simulink model "VCMGCM1962020b_v2"  (R2020b)
settings: Solver=FixedStepDiscrete  StartTime=0.0  StopTime=10.0  FixedStep=0.005  RelTol=1e-3  EnableMultiTasking=on
PreLoadFcn:
  | try, model_open; catch, disp('Error occurred while executing model pre-load callback: model_open.m'); disp('Please assure that the MATLAB working directory is set to the model directory before opening.'); end
InitFcn:
  | try, model_open; catch, end
undefined symbols (not defined in the file): Bridge, GCM, H, raptor_get_param_eval, raptor_get_safe_string, raptor_xcp_function
libraries: Blocks_lib x1165, Raptor_lib x665, simulink x62, VCM_lib x5
(part 13 of 23)

== system VCMGCM1962020b_v2/Fgnd/Sensors/CAN/DC//DC Converter/DCDC_Status_0_16V ==
  DiagEnbl : Inport
  Bus Creator : BusCreator  Inputs=7
  CANRxField1 : Blocks_lib/CANRxField  typ='uint8'  custom=off  custom_nam=[nam '---']  custom_units='---'
  CANRxField2 : Blocks_lib/CANRxField  typ='double'  custom=off  custom_nam=[nam '---']  custom_units='---'
  CANRxField3 : Blocks_lib/CANRxField  typ='double'  custom=off  custom_nam=[nam '---']  custom_units='---'
  CANRxField4 : Blocks_lib/CANRxField  typ='uint16'  custom=off  custom_nam=[nam '---']  custom_units='---'
  CANRxField5 : Blocks_lib/CANRxField  typ='boolean'  custom=off  custom_nam=[nam '---']  custom_units='---'
  CANRxField6 : Blocks_lib/CANRxField  typ='double'  custom=off  custom_nam=[nam '---']  custom_units='---'
  CANRxMsgStatus : Blocks_lib/CANRxMsgStatus  samptime=samptime  custom=off  custom_nam=['---']  msgnam=DCDC_Status_0_16V
  Header : Blocks_lib/Header  width=Landscape  addtext=''
  raptor_can_rxmsg : Raptor_lib/CAN/raptor_can_rxmsg  canDefinition=struct('dbcFile', 'Dilong DCDC Converter_dbc file_v2.dbc','message', 'DCDC_Status_0_16V','comment', '','signals', {{'Fault_alarm2_0_16V','Fault_alarm1_0_16V','DCDC_Output_Current_0_16V','DCDCOutput_Voltage_0_16V','DCDC_Run_status_0_16V','DCDC_Inner_temp_0_16V'}},'enabled', [ 1 1 1 1 1 1;],'scaled', [ 1 1 1 1 1 1;],'canBus', 'bus','messageID', [ 402712053;],'idMask', [ 536870911;],'payloadMask', [],'payloadValue', [],'period', [ 0;],'mailbox', '''''','queueSize', [ 1;],'label', [ 1;],'ver', [ 2;],'showID', [ 0;],'showRaw', [ 0;],'fill', [ 0;],'editID', [ 0;],'signalOrder', [ 3;],'signalAscDes', [ 1;])  canBus=bus  mailbox=''  payloadMask=[]  payloadValue=[]  idMask=hex2dec('1FFFFFFF')  queueSize=1  showID=0  label=1  fill=0  id=402712053  showRaw=0  showAge=1  signalOrder=3  signalInfo={{struct('Name', 'Fault_alarm2_0_16V','Startbit', [ 0;],'SignalSize', [ 8;],'ByteOrder', 'LittleEndian','ValueType', 'UNSIGNED','Class', 'uint8','Signed', [ 0;],'Factor', [ 1;],'Offset', [ 0;],'Min', [ 0;],'Max', [ 128;],'Units', '','Comment', '','StartBit', [ 8;]),struct('Name', 'Fault_alarm1_0_16V','Startbit', [ 0;],'SignalSize', [ 8;],'ByteOrder', 'LittleEndian','ValueType', 'UNSIGNED','Class', 'uint8','Signed', [ 0;],'Factor', [ 1;],'Offset', [ 0;],'Min', [ 0;],'Max', [ 128;],'Units', '','Comment', '','StartBit', [ 16;]),struct('Name', 'DCDC_Output_Current_0_16V','Startbit', [ 0;],'SignalSize', [ 16;],'ByteOrder', 'LittleEndian','ValueType', 'UNSIGNED','Class', 'uint16','Signed', [ 0;],'Factor', [ 0.1;],'Offset', [ 0;],'Min', [ 0;],'Max', [ 1500;],'Units', 'A','Comment', '','StartBit', [ 24;]),struct('Name', 'DCDCOutput_Voltage_0_16V','Startbit', [ 0;],'SignalSize', [ 8;],'ByteOrder', 'LittleEndian','ValueType', 'UNSIGNED','Class', 'uint8','Signed', [ 0;],'Factor', [ 0.2;],'Offset', [ 0;],'Min', [ 0;],'Max', [ 150;],'Units', 'V','Comment', '','StartBit', [ 40;]),struct('Name', 'DCDC_Run_status_0_16V','Startbit', [ 0;],'SignalSize', [ 1;],'ByteOrder', 'LittleEndian','ValueType', 'UNSIGNED','Class', 'uint8','Signed', [ 0;],'Factor', [ 1;],'Offset', [ 0;],'Min', [ 0;],'Max', [ 1;],'Units', '','Comment', '','StartBit', [ 48;]),struct('Name', 'DCDC_Inner_temp_0_16V','Startbit', [ 0;],'SignalSize', [ 8;],'ByteOrder', 'LittleEndian','ValueType', 'UNSIGNED','Class', 'uint8','Signed', [ 0;],'Factor', [ 1;],'Offset', [ -40;],'Min', [ 0;],'Max', [ 128;],'Units', 'C','Comment', '','StartBit', [ 56;])}}
      settings: SourceProductName=Raptor
  Data : Outport  VectorParamsAs1DForOutWhenUnconnected=off
  wires:
  Bus Creator/1 -> Data/1  "DCDC_Status_0_16V"
  raptor_can_rxmsg/2 -> CANRxField4/1  "Fault_alarm2_0_16V"
  raptor_can_rxmsg/3 -> CANRxField1/1  "Fault_alarm1_0_16V"
  raptor_can_rxmsg/4 -> CANRxField3/1  "DCDC_Output_Current_0_16V"
  DiagEnbl/1 -> CANRxMsgStatus/1
  raptor_can_rxmsg/1 -> CANRxMsgStatus/2  "Age"
  CANRxMsgStatus/1 -> Bus Creator/1
  CANRxField4/1 -> Bus Creator/2
  CANRxField1/1 -> Bus Creator/3
  CANRxField3/1 -> Bus Creator/4
  CANRxField2/1 -> Bus Creator/7
  raptor_can_rxmsg/7 -> CANRxField2/1  "DCDC_Inner_temp_0_16V"
  raptor_can_rxmsg/6 -> CANRxField5/1  "DCDC_Run_status_0_16V"
  raptor_can_rxmsg/5 -> CANRxField6/1  "DCDCOutput_Voltage_0_16V"
  CANRxField5/1 -> Bus Creator/6
  CANRxField6/1 -> Bus Creator/5

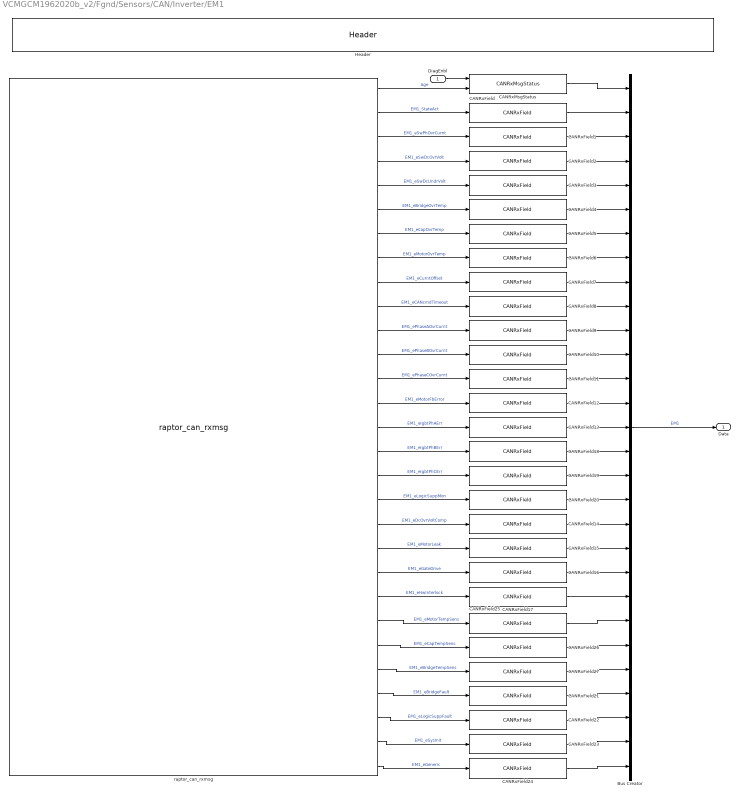
== system VCMGCM1962020b_v2/Fgnd/Sensors/CAN/Inverter/EM1 ==
  DiagEnbl : Inport
  Bus Creator : BusCreator  Inputs=29
  CANRxField : Blocks_lib/CANRxField  typ='uint8'  custom=off  custom_nam='---'  custom_units='---'
  CANRxField{1..24,26..27} (26 alike) : Blocks_lib/CANRxField  typ='boolean'  custom=off  custom_nam='---'  custom_units='---'
  CANRxField25 : Blocks_lib/CANRxField  typ='uint8'  custom=off  custom_nam='---'  custom_units='---'
  CANRxMsgStatus : Blocks_lib/CANRxMsgStatus  samptime=samptime  custom=off  custom_nam='Name'  msgnam=EM1
  Header : Blocks_lib/Header  width=Landscape  addtext=''
  raptor_can_rxmsg : Raptor_lib/CAN/raptor_can_rxmsg  canDefinition=struct('dbcFile', '20220526e_emDrive_NodeID_0x01.dbc','message', 'EM1','comment', '100ms','signals', {{'EM1_StateAct','EM1_eSwPhOvrCurnt','EM1_eSwDcOvrVolt','EM1_eSwDcUndrVolt','EM1_eBridgeOvrTemp','EM1_eCapOvrTemp','EM1_eMotorOvrTemp','EM1_eCurntOffset','EM1_eCANcmdTimeout','EM1_ePhaseAOvrCurnt','EM1_ePhaseBOvrCurnt','EM1_ePhaseCOvrCurnt','EM1_eMotorFbError','EM1_eIgbtPhAErr','EM1_eIgbtPhBErr','EM1_eIgbtPhCErr','EM1_eLogicSuppMon','EM1_eDcOvrVoltComp','EM1_eMotorLeak','EM1_eGateDrive','EM1_eHwInterlock','EM1_eMotorTempSens','EM1_eCapTempSens','EM1_eBridgeTempSens','EM1_eBridgeFault','EM1_eLogicSuppFault','EM1_eSysInit','EM1_eGeneric'}},'enabled', [ 1 1 1 1 1 1 1 1 1 1 1 1 1 1 1 1 1 1 1 1 1 1 1 1 1 1 1 1;],'scaled', [ 1 1 1 1 1 1 1 1 1 1 1 1 1 1 1 1 1 1 1 1 1 1 1 1 1 1 1 1;],'canBus', 'bus','messageID', [ 385;],'idMask', [ 536870911;],'payloadMask', [],'payloadValue', [],'period', [ 0;],'mailbox', '''''','queueSize', [ 1;],'label', [ 1;],'ver', [ 2;],'showID', [ 0;],'showRaw', [ 0;],'showRawMsg', [ 0;],'showAge', [ 1;],'fill', [ 0;],'editID', [ 0;],'signalOrder', [ 3;],'signalAscDes', [ 1;])  canBus=bus  mailbox=''  payloadMask=[]  payloadValue=[]  idMask=hex2dec('1FFFFFFF')  queueSize=1  showID=0  label=1  fill=0  id=385  showRaw=0  showAge=1  signalOrder=3  signalInfo={{struct('Name', 'EM1_StateAct','Startbit', [ 0;],'SignalSize', [ 8;],'ByteOrder', 'LittleEndian','ValueType', 'UNSIGNED','Class', 'uint8','Signed', [ 0;],'Factor', [ 1;],'Offset', [ 0;],'Min', [ -2;],'Max', [ 2;],'Units', '','Comment', 'Application_Control__State','StartBit', [ 0;]),struct('Name', 'EM1_eSwPhOvrCurnt','Startbit', [ 0;],'SignalSize', [ 1;],'ByteOrder', 'LittleEndian','ValueType', 'UNSIGNED','Class', 'uint8','Signed', [ 0;],'Factor', [ 1;],'Offset', [ 0;],'Min', [ 0;],'Max', [ 1;],'Units', '','Comment', 'Software phase overcurrent','StartBit', [ 8;]),struct('Name', 'EM1_eSwDcOvrVolt','Startbit', [ 0;],'SignalSize', [ 1;],'ByteOrder', 'LittleEndian','ValueType', 'UNSIGNED','Class', 'uint8','Signed', [ 0;],'Factor', [ 1;],'Offset', [ 0;],'Min', [ 0;],'Max', [ 1;],'Units', '','Comment', 'Software DC link overvoltage','StartBit', [ 9;]),struct('Name', 'EM1_eSwDcUndrVolt','Startbit', [ 0;],'SignalSize', [ 1;],'ByteOrder', 'LittleEndian','ValueType', 'UNSIGNED','Class', 'uint8','Signed', [ 0;],'Factor', [ 1;],'Offset', [ 0;],'Min', [ 0;],'Max', [ 1;],'Units', '','Comment', 'Software DC link undervoltage','StartBit', [ 10;]),struct('Name', 'EM1_eBridgeOvrTemp','Startbit', [ 0;],'SignalSize', [ 1;],'ByteOrder', 'LittleEndian','ValueType', 'UNSIGNED','Class', 'uint8','Signed', [ 0;],'Factor', [ 1;],'Offset', [ 0;],'Min', [ 0;],'Max', [ 1;],'Units', '','Comment', 'Bridge overtemperature','StartBit', [ 11;]),struct('Name', 'EM1_eCapOvrTemp','Startbit', [ 0;],'SignalSize', [ 1;],'ByteOrder', 'LittleEndian','ValueType', 'UNSIGNED','Class', 'uint8','Signed', [ 0;],'Factor', [ 1;],'Offset', [ 0;],'Min', [ 0;],'Max', [ 1;],'Units', '','Comment', 'Capacitor overtemperature','StartBit', [ 12;]),struct('Name', 'EM1_eMotorOvrTemp','Startbit', [ 0;],'SignalSize', [ 1;],'ByteOrder', 'LittleEndian','ValueType', 'UNSIGNED','Class', 'uint8','Signed', [ 0;],'Factor', [ 1;],'Offset', [ 0;],'Min', [ 0;],'Max', [ 1;],'Units', '','Comment', 'Motor overtemperature','StartBit', [ 13;]),struct('Name', 'EM1_eCurntOffset','Startbit', [ 0;],'SignalSize', [ 1;],'ByteOrder', 'LittleEndian','ValueType', 'UNSIGNED','Class', 'uint8','Signed', [ 0;],'Factor', [ 1;],'Offset', [ 0;],'Min', [ 0;],'Max', [ 1;],'Units', '','Comment', 'Current offset','StartBit', [ 14;]),struct('Name', 'EM1_eCANcmdTimeout','Startbit', [ 0;],'SignalSize', [ 1;],'ByteOrder', 'LittleEndian','ValueType', 'UNSIGNED','Class', 'uint8','Signed', [ 0;],'Factor', [ 1;],'Offset', [ 0;],'Min', [ 0;],'Max', [ 1;],'Units', '','Comment', 'CAN Command timeout','StartBit', [ 15;]),struct('Name', 'EM1_ePhaseAOvrCurnt','Startbit', [ 0;],'SignalSize', [ 1;],'ByteOrder', 'LittleEndian','ValueType', 'UNSIGNED','Class', 'uint8','Signed', [ 0;],'Factor', [ 1;],'Offset', [ 0;],'Min', [ 0;],'Max', [ 1;],'Units', '','Comment', 'Phase A overcurrent','StartBit', [ 16;]),struct('Name', 'EM1_ePhaseBOvrCurnt','Startbit', [ 0;],'SignalSize', [ 1;],'ByteOrder', 'LittleEndian','ValueType', 'UNSIGNED','Class', 'uint8','Signed', [ 0;],'Factor', [ 1;],'Offset', [ 0;],'Min', [ 0;],'Max', [ 1;],'Units', '','Comment', 'Phase B overcurrent','StartBit', [ 17;]),struct('Name', 'EM1_ePhaseCOvrCurnt','Startbit', [ 0;],'SignalSize', [ 1;],'ByteOrder', 'LittleEndian','ValueType', 'UNSIGNED','Class', 'uint8','Signed', [ 0;],'Factor', [ 1;],'Offset', [ 0;],'Min', [ 0;],'Max', [ 1;],'Units', '','Comment', 'Phase C overcurrent','StartBit', [ 18;]),struct('Name', 'EM1_eMotorFbError','Startbit', [ 0;],'SignalSize', [ 1;],'ByteOrder', 'LittleEndian','ValueType', 'UNSIGNED','Class', 'uint8','Signed', [ 0;],'Factor', [ 1;],'Offset', [ 0;],'Min', [ 0;],'Max', [ 1;],'Units', '','Comment', 'Motor feedback error','StartBit', [ 19;]),struct('Name', 'EM1_eIgbtPhAErr','Startbit', [ 0;],'SignalSize', [ 1;],'ByteOrder', 'LittleEndian','ValueType', 'UNSIGNED','Class', 'uint8','Signed', [ 0;],'Factor', [ 1;],'Offset', [ 0;],'Min', [ 0;],'Max', [ 1;],'Units', '','Comment', 'IGBT Phase A error','StartBit', [ 20;]),struct('Name', 'EM1_eIgbtPhBErr','Startbit', [ 0;],'SignalSize', [ 1;],'ByteOrder', 'LittleEndian','ValueType', 'UNSIGNED','Class', 'uint8','Signed', [ 0;],'Factor', [ 1;],'Offset', [ 0;],'Min', [ 0;],'Max', [ 1;],'Units', '','Comment', 'IGBT Phase B error','StartBit', [ 21;]),struct('Name', 'EM1_eIgbtPhCErr','Startbit', [ 0;],'SignalSize', [ 1;],'ByteOrder', 'LittleEndian','ValueType', 'UNSIGNED','Class', 'uint8','Signed', [ 0;],'Factor', [ 1;],'Offset', [ 0;],'Min', [ 0;],'Max', [ 1;],'Units', '','Comment', 'IGBT Phase C error','StartBit', [ 22;]),struct('Name', 'EM1_eLogicSuppMon','Startbit', [ 0;],'SignalSize', [ 1;],'ByteOrder', 'LittleEndian','ValueType', 'UNSIGNED','Class', 'uint8','Signed', [ 0;],'Factor', [ 1;],'Offset', [ 0;],'Min', [ 0;],'Max', [ 1;],'Units', '','Comment', 'Logic Supply monitor error','StartBit', [ 24;]),struct('Name', 'EM1_eDcOvrVoltComp','Startbit', [ 0;],'SignalSize', [ 1;],'ByteOrder', 'LittleEndian','ValueType', 'UNSIGNED','Class', 'uint8','Signed', [ 0;],'Factor', [ 1;],'Offset', [ 0;],'Min', [ 0;],'Max', [ 1;],'Units', '','Comment', 'DC link overvoltage comparator','StartBit', [ 25;]),struct('Name', 'EM1_eMotorLeak','Startbit', [ 0;],'SignalSize', [ 1;],'ByteOrder', 'LittleEndian','ValueType', 'UNSIGNED','Class', 'uint8','Signed', [ 0;],'Factor', [ 1;],'Offset', [ 0;],'Min', [ 0;],'Max', [ 1;],'Units', '','Comment', 'Motor leakage','StartBit', [ 26;]),struct('Name', 'EM1_eGateDrive','Startbit', [ 0;],'SignalSize', [ 1;],'ByteOrder', 'LittleEndian','ValueType', 'UNSIGNED','Class', 'uint8','Signed', [ 0;],'Factor', [ 1;],'Offset', [ 0;],'Min', [ 0;],'Max', [ 1;],'Units', '','Comment', 'Gatedriver error','StartBit', [ 27;]),struct('Name', 'EM1_eHwInterlock','Startbit', [ 0;],'SignalSize', [ 1;],'ByteOrder', 'LittleEndian','ValueType', 'UNSIGNED','Class', 'uint8','Signed', [ 0;],'Factor', [ 1;],'Offset', [ 0;],'Min', [ 0;],'Max', [ 1;],'Units', '','Comment', 'HW interlock','StartBit', [ 28;]),struct('Name', 'EM1_eMotorTempSens','Startbit', [ 0;],'SignalSize', [ 1;],'ByteOrder', 'LittleEndian','ValueType', 'UNSIGNED','Class', 'uint8','Signed', [ 0;],'Factor', [ 1;],'Offset', [ 0;],'Min', [ 0;],'Max', [ 1;],'Units', '','Comment', 'Motor temperature sensor fail','StartBit', [ 29;]),struct('Name', 'EM1_eCapTempSens','Startbit', [ 0;],'SignalSize', [ 1;],'ByteOrder', 'LittleEndian','ValueType', 'UNSIGNED','Class', 'uint8','Signed', [ 0;],'Factor', [ 1;],'Offset', [ 0;],'Min', [ 0;],'Max', [ 1;],'Units', '','Comment', 'Capacitor temperature sensor fail','StartBit', [ 30;]),struct('Name', 'EM1_eBridgeTempSens','Startbit', [ 0;],'SignalSize', [ 1;],'ByteOrder', 'LittleEndian','ValueType', 'UNSIGNED','Class', 'uint8','Signed', [ 0;],'Factor', [ 1;],'Offset', [ 0;],'Min', [ 0;],'Max', [ 1;],'Units', '','Comment', 'Bridge temperature sensor fail','StartBit', [ 31;]),struct('Name', 'EM1_eBridgeFault','Startbit', [ 0;],'SignalSize', [ 1;],'ByteOrder', 'LittleEndian','ValueType', 'UNSIGNED','Class', 'uint8','Signed', [ 0;],'Factor', [ 1;],'Offset', [ 0;],'Min', [ 0;],'Max', [ 1;],'Units', '','Comment', 'Bridge fault (check BridgeFault object for details)','StartBit', [ 32;]),struct('Name', 'EM1_eLogicSuppFault','Startbit', [ 0;],'SignalSize', [ 1;],'ByteOrder', 'LittleEndian','ValueType', 'UNSIGNED','Class', 'uint8','Signed', [ 0;],'Factor', [ 1;],'Offset', [ 0;],'Min', [ 0;],'Max', [ 1;],'Units', '','Comment', 'Logic supply fault','StartBit', [ 33;]),struct('Name', 'EM1_eSysInit','Startbit', [ 0;],'SignalSize', [ 1;],'ByteOrder', 'LittleEndian','ValueType', 'UNSIGNED','Class', 'uint8','Signed', [ 0;],'Factor', [ 1;],'Offset', [ 0;],'Min', [ 0;],'Max', [ 1;],'Units', '','Comment', 'System initialization error','StartBit', [ 38;]),struct('Name', 'EM1_eGeneric','Startbit', [ 0;],'SignalSize', [ 1;],'ByteOrder', 'LittleEndian','ValueType', 'UNSIGNED','Class', 'uint8','Signed', [ 0;],'Factor', [ 1;],'Offset', [ 0;],'Min', [ 0;],'Max', [ 1;],'Units', '','Comment', 'Generic error','StartBit', [ 39;])}}
      settings: SourceProductName=Raptor
  Data : Outport  VectorParamsAs1DForOutWhenUnconnected=off
  wires:
  Bus Creator/1 -> Data/1  "EM1"
  raptor_can_rxmsg/2 -> CANRxField/1  "EM1_StateAct"
  CANRxMsgStatus/1 -> Bus Creator/1
  DiagEnbl/1 -> CANRxMsgStatus/1
  raptor_can_rxmsg/1 -> CANRxMsgStatus/2  "Age"
  raptor_can_rxmsg/3 -> CANRxField1/1  "EM1_eSwPhOvrCurnt"
  raptor_can_rxmsg/4 -> CANRxField2/1  "EM1_eSwDcOvrVolt"
  raptor_can_rxmsg/5 -> CANRxField3/1  "EM1_eSwDcUndrVolt"
  raptor_can_rxmsg/6 -> CANRxField4/1  "EM1_eBridgeOvrTemp"
  raptor_can_rxmsg/7 -> CANRxField5/1  "EM1_eCapOvrTemp"
  raptor_can_rxmsg/8 -> CANRxField6/1  "EM1_eMotorOvrTemp"
  raptor_can_rxmsg/9 -> CANRxField7/1  "EM1_eCurntOffset"
  raptor_can_rxmsg/10 -> CANRxField8/1  "EM1_eCANcmdTimeout"
  raptor_can_rxmsg/11 -> CANRxField9/1  "EM1_ePhaseAOvrCurnt"
  raptor_can_rxmsg/12 -> CANRxField10/1  "EM1_ePhaseBOvrCurnt"
  raptor_can_rxmsg/13 -> CANRxField11/1  "EM1_ePhaseCOvrCurnt"
  raptor_can_rxmsg/14 -> CANRxField12/1  "EM1_eMotorFbError"
  raptor_can_rxmsg/15 -> CANRxField13/1  "EM1_eIgbtPhAErr"
  raptor_can_rxmsg/16 -> CANRxField18/1  "EM1_eIgbtPhBErr"
  raptor_can_rxmsg/17 -> CANRxField19/1  "EM1_eIgbtPhCErr"
  raptor_can_rxmsg/18 -> CANRxField20/1  "EM1_eLogicSuppMon"
  raptor_can_rxmsg/19 -> CANRxField14/1  "EM1_eDcOvrVoltComp"
  raptor_can_rxmsg/20 -> CANRxField15/1  "EM1_eMotorLeak"
  raptor_can_rxmsg/21 -> CANRxField16/1  "EM1_eGateDrive"
  raptor_can_rxmsg/22 -> CANRxField17/1  "EM1_eHwInterlock"
  raptor_can_rxmsg/23 -> CANRxField25/1  "EM1_eMotorTempSens"
  raptor_can_rxmsg/24 -> CANRxField26/1  "EM1_eCapTempSens"
  raptor_can_rxmsg/25 -> CANRxField27/1  "EM1_eBridgeTempSens"
  raptor_can_rxmsg/26 -> CANRxField21/1  "EM1_eBridgeFault"
  raptor_can_rxmsg/27 -> CANRxField22/1  "EM1_eLogicSuppFault"
  raptor_can_rxmsg/28 -> CANRxField23/1  "EM1_eSysInit"
  raptor_can_rxmsg/29 -> CANRxField24/1  "EM1_eGeneric"
  CANRxField/1 -> Bus Creator/2
  CANRxField1/1 -> Bus Creator/3
  CANRxField2/1 -> Bus Creator/4
  CANRxField3/1 -> Bus Creator/5
  CANRxField4/1 -> Bus Creator/6
  CANRxField5/1 -> Bus Creator/7
  CANRxField6/1 -> Bus Creator/8
  CANRxField7/1 -> Bus Creator/9
  CANRxField8/1 -> Bus Creator/10
  CANRxField9/1 -> Bus Creator/11
  CANRxField10/1 -> Bus Creator/12
  CANRxField11/1 -> Bus Creator/13
  CANRxField12/1 -> Bus Creator/14
  CANRxField13/1 -> Bus Creator/15
  CANRxField18/1 -> Bus Creator/16
  CANRxField19/1 -> Bus Creator/17
  CANRxField20/1 -> Bus Creator/18
  CANRxField14/1 -> Bus Creator/19
  CANRxField15/1 -> Bus Creator/20
  CANRxField16/1 -> Bus Creator/21
  CANRxField17/1 -> Bus Creator/22
  CANRxField25/1 -> Bus Creator/23
  CANRxField26/1 -> Bus Creator/24
  CANRxField27/1 -> Bus Creator/25
  CANRxField21/1 -> Bus Creator/26
  CANRxField22/1 -> Bus Creator/27
  CANRxField23/1 -> Bus Creator/28
  CANRxField24/1 -> Bus Creator/29

== system VCMGCM1962020b_v2/Fgnd/Sensors/CAN/Inverter/EM2_InvTemp ==
  note: This is a CANR Rx structure that was implemented to overcome a error in the way the floating point data was handled. It is not Ideal but does work.
  DiagEnbl : Inport
  Bus Creator1 : BusCreator  Inputs=2
  Bus Creator2 : BusCreator  Inputs=2
  Bus Creator3 : BusCreator  Inputs=2
  Delay : Delay  DelayLength=5
  EM2InvTemp : Subsystem
  EM2MtrTemp : Subsystem
  Header : Blocks_lib/Header  width=Landscape  addtext=''
  NOT : Logic  Operator=NOT  AllPortsSameDT=off  OutDataTypeStr=boolean
  Output : Outport
  wires:
  EM2MtrTemp/1(MsgVld) -> Bus Creator2/1
  EM2MtrTemp/2(Out2) -> Bus Creator2/2
  DiagEnbl/1 -> EM2MtrTemp/1(DiagEnbl), EM2InvTemp/1(DiagEnbl)
  Bus Creator2/1 -> Bus Creator1/2  "EM2MtrTemp"
  Delay/1 -> NOT/1, EM2InvTemp/Enable
  NOT/1 -> Delay/1, EM2MtrTemp/Enable
  Bus Creator1/1 -> Output/1  "EM2"
  EM2InvTemp/1(MsgVld) -> Bus Creator3/1
  EM2InvTemp/2(Out2) -> Bus Creator3/2
  Bus Creator3/1 -> Bus Creator1/1  "EM2Invemp"

== system VCMGCM1962020b_v2/Fgnd/Sensors/CAN/Inverter/EM3 ==
  DiagEnbl : Inport
  Bus Creator : BusCreator  Inputs=3
  CANRxField : Blocks_lib/CANRxField  typ='double'  custom=off  custom_nam='---'  custom_units='---'
  CANRxField1 : Blocks_lib/CANRxField  typ='double'  custom=off  custom_nam='---'  custom_units='---'
  CANRxMsgStatus : Blocks_lib/CANRxMsgStatus  samptime=samptime  custom=off  custom_nam='Name'  msgnam=EM3
  Header : Blocks_lib/Header  width=Landscape  addtext=''
  raptor_can_rxmsg : Raptor_lib/CAN/raptor_can_rxmsg  canDefinition=struct('dbcFile', '20220526e_emDrive_NodeID_0x01.dbc','message', 'EM3','comment', '40ms','signals', {{'EM3_InverterDcV','EM3_PhaseAmpsRms'}},'enabled', [ 1 1;],'scaled', [ 1 1;],'canBus', 'bus','messageID', [ 897;],'idMask', [ 536870911;],'payloadMask', [],'payloadValue', [],'period', [ 0;],'mailbox', '''''','queueSize', [ 1;],'label', [ 1;],'ver', [ 2;],'showID', [ 0;],'showRaw', [ 0;],'fill', [ 0;],'editID', [ 0;],'signalOrder', [ 3;],'signalAscDes', [ 1;])  canBus=bus  mailbox=''  payloadMask=[]  payloadValue=[]  idMask=hex2dec('1FFFFFFF')  queueSize=1  showID=0  label=1  fill=0  id=897  showRaw=0  showAge=1  signalOrder=3  signalInfo={{struct('Name', 'EM3_InverterDcV','Startbit', [ 0;],'SignalSize', [ 32;],'ByteOrder', 'LittleEndian','ValueType', 'FLOAT32','Class', 'single','Signed', [ 1;],'Factor', [ 1;],'Offset', [ 0;],'Min', [ 0;],'Max', [ 0;],'Units', 'V','Comment', 'HW_Monitor__UDC','StartBit', [ 0;]),struct('Name', 'EM3_PhaseAmpsRms','Startbit', [ 0;],'SignalSize', [ 32;],'ByteOrder', 'LittleEndian','ValueType', 'FLOAT32','Class', 'single','Signed', [ 1;],'Factor', [ 1;],'Offset', [ 0;],'Min', [ 0;],'Max', [ 0;],'Units', 'A','Comment', 'HW_Monitor__Phase_Current','StartBit', [ 32;])}}
      settings: SourceProductName=Raptor
  Data : Outport  VectorParamsAs1DForOutWhenUnconnected=off
  wires:
  Bus Creator/1 -> Data/1  "MsgName"
  raptor_can_rxmsg/2 -> CANRxField/1  "EM3_InverterDcV"
  CANRxMsgStatus/1 -> Bus Creator/1
  DiagEnbl/1 -> CANRxMsgStatus/1
  raptor_can_rxmsg/1 -> CANRxMsgStatus/2  "Age"
  CANRxField/1 -> Bus Creator/2
  raptor_can_rxmsg/3 -> CANRxField1/1  "EM3_PhaseAmpsRms"
  CANRxField1/1 -> Bus Creator/3

== system VCMGCM1962020b_v2/Fgnd/Sensors/CAN/Inverter/EM3_DCV ==
  note: This is a CANR Rx structure that was implemented to overcome a error in the way the floating point data was handled. It is not Ideal but does work.
  DiagEnbl : Inport
  Bus Creator1 : BusCreator  Inputs=2
  Bus Creator2 : BusCreator  Inputs=2
  Bus Creator3 : BusCreator  Inputs=2
  Delay : Delay  DelayLength=5
  EM3DCv : Subsystem
  EM3PhCur : Subsystem
  Header : Blocks_lib/Header  width=Landscape  addtext=''
  NOT : Logic  Operator=NOT  AllPortsSameDT=off  OutDataTypeStr=boolean
  Output : Outport
  wires:
  EM3PhCur/1(MsgVld) -> Bus Creator2/1
  EM3PhCur/2(Out2) -> Bus Creator2/2
  DiagEnbl/1 -> EM3PhCur/1(DiagEnbl), EM3DCv/1(DiagEnbl)
  Bus Creator2/1 -> Bus Creator1/2  "EM3PhCur"
  Delay/1 -> NOT/1, EM3DCv/Enable
  NOT/1 -> Delay/1, EM3PhCur/Enable
  Bus Creator1/1 -> Output/1  "EM3"
  EM3DCv/1(MsgVld) -> Bus Creator3/1
  EM3DCv/2(Out2) -> Bus Creator3/2
  Bus Creator3/1 -> Bus Creator1/1  "EM3DCv"

== system VCMGCM1962020b_v2/Fgnd/Sensors/CAN/Inverter/EM4 ==
  DiagEnbl : Inport
  Bus Creator : BusCreator  Inputs=3
  CANRxField : Blocks_lib/CANRxField  typ='double'  custom=off  custom_nam='---'  custom_units='---'
  CANRxField1 : Blocks_lib/CANRxField  typ='double'  custom=off  custom_nam='---'  custom_units='---'
  CANRxMsgStatus : Blocks_lib/CANRxMsgStatus  samptime=samptime  custom=off  custom_nam='Name'  msgnam=EM4
  Header : Blocks_lib/Header  width=Landscape  addtext=''
  raptor_can_rxmsg : Raptor_lib/CAN/raptor_can_rxmsg  canDefinition=struct('dbcFile', '20220526e_emDrive_NodeID_0x01.dbc','message', 'EM4','comment', '20ms','signals', {{'EM4_TorqAct','EM4_SpdAct'}},'enabled', [ 1 1;],'scaled', [ 1 1;],'canBus', 'bus','messageID', [ 641;],'idMask', [ 536870911;],'payloadMask', [],'payloadValue', [],'period', [ 0;],'mailbox', '''''','queueSize', [ 1;],'label', [ 1;],'ver', [ 2;],'showID', [ 0;],'showRaw', [ 0;],'fill', [ 0;],'editID', [ 0;],'signalOrder', [ 3;],'signalAscDes', [ 1;])  canBus=bus  mailbox=''  payloadMask=[]  payloadValue=[]  idMask=hex2dec('1FFFFFFF')  queueSize=1  showID=0  label=1  fill=0  id=641  showRaw=0  showAge=1  signalOrder=3  signalInfo={{struct('Name', 'EM4_TorqAct','Startbit', [ 0;],'SignalSize', [ 32;],'ByteOrder', 'LittleEndian','ValueType', 'FLOAT32','Class', 'single','Signed', [ 1;],'Factor', [ 1;],'Offset', [ 0;],'Min', [ 0;],'Max', [ 0;],'Units', 'Nm','Comment', 'Ctrl_Gen_Stat__Tact','StartBit', [ 0;]),struct('Name', 'EM4_SpdAct','Startbit', [ 0;],'SignalSize', [ 32;],'ByteOrder', 'LittleEndian','ValueType', 'FLOAT32','Class', 'single','Signed', [ 1;],'Factor', [ 1;],'Offset', [ 0;],'Min', [ 0;],'Max', [ 0;],'Units', 'rpm','Comment', 'Ctrl_Gen_Stat__RPMact','StartBit', [ 32;])}}
      settings: SourceProductName=Raptor
  Data : Outport  VectorParamsAs1DForOutWhenUnconnected=off
  wires:
  CANRxField/1 -> Bus Creator/2
  raptor_can_rxmsg/1 -> CANRxMsgStatus/2  "Age"
  DiagEnbl/1 -> CANRxMsgStatus/1
  CANRxMsgStatus/1 -> Bus Creator/1
  raptor_can_rxmsg/2 -> CANRxField/1  "EM4_TorqAct"
  Bus Creator/1 -> Data/1  "MsgName"
  raptor_can_rxmsg/3 -> CANRxField1/1  "EM4_SpdAct"
  CANRxField1/1 -> Bus Creator/3

== system VCMGCM1962020b_v2/Fgnd/Sensors/CAN/Inverter/EM4_Spd ==
  note: This is a CANR Rx structure that was implemented to overcome a error in the way the floating point data was handled. It is not Ideal but does work.
  DiagEnbl : Inport
  Bus Creator1 : BusCreator  Inputs=2
  Bus Creator2 : BusCreator  Inputs=2
  Bus Creator3 : BusCreator  Inputs=2
  Delay : Delay
  EM4Spd : Subsystem
  EM4Torq : Subsystem
  Header : Blocks_lib/Header  width=Landscape  addtext=''
  NOT : Logic  Operator=NOT  AllPortsSameDT=off  OutDataTypeStr=boolean
  Output : Outport
  wires:
  EM4Torq/1(MsgVld) -> Bus Creator2/1
  EM4Torq/2(Out2) -> Bus Creator2/2
  DiagEnbl/1 -> EM4Torq/1(DiagEnbl), EM4Spd/1(DiagEnbl)
  Bus Creator2/1 -> Bus Creator1/2  "EM4Trq"
  Delay/1 -> NOT/1, EM4Spd/Enable
  NOT/1 -> Delay/1, EM4Torq/Enable
  Bus Creator1/1 -> Output/1  "EM4"
  EM4Spd/1(MsgVld) -> Bus Creator3/1
  EM4Spd/2(Out2) -> Bus Creator3/2
  Bus Creator3/1 -> Bus Creator1/1  "EM4Spd"

== system VCMGCM1962020b_v2/Fgnd/Sensors/CAN/Inverter/EM_BOOT ==
  DiagEnbl : Inport
  Bus Creator : BusCreator  Inputs=2
  CANRxField : Blocks_lib/CANRxField  typ='double'  custom=off  custom_nam='---'  custom_units='---'
  CANRxMsgStatus : Blocks_lib/CANRxMsgStatus  samptime=samptime  custom=off  custom_nam='Name'  msgnam=EM_BOOT
  Header : Blocks_lib/Header  width=Landscape  addtext=''
  raptor_can_rxmsg : Raptor_lib/CAN/raptor_can_rxmsg  canDefinition=struct('dbcFile', '20220526e_emDrive_NodeID_0x01.dbc','message', 'EM_BOOT','comment', 'Sent after boot has completed and comms are available','signals', {{'EM_BOOT_EmBoot'}},'enabled', [ 1;],'scaled', [ 1;],'canBus', 'bus','messageID', [ 1793;],'idMask', [ 536870911;],'payloadMask', [],'payloadValue', [],'period', [ 0;],'mailbox', '''''','queueSize', [ 1;],'label', [ 1;],'ver', [ 2;],'showID', [ 0;],'showRaw', [ 0;],'showRawMsg', [ 0;],'showAge', [ 1;],'fill', [ 0;],'editID', [ 0;],'signalOrder', [ 3;],'signalAscDes', [ 1;])  canBus=bus  mailbox=''  payloadMask=[]  payloadValue=[]  idMask=hex2dec('1FFFFFFF')  queueSize=1  showID=0  label=1  fill=0  id=1793  showRaw=0  showAge=1  signalOrder=3  signalInfo={{struct('Name', 'EM_BOOT_EmBoot','Startbit', [ 0;],'SignalSize', [ 8;],'ByteOrder', 'LittleEndian','ValueType', 'UNSIGNED','Class', 'uint8','Signed', [ 0;],'Factor', [ 1;],'Offset', [ 0;],'Min', [ 0;],'Max', [ 0;],'Units', '','Comment', '','StartBit', [ 0;])}}
      settings: SourceProductName=Raptor
  Data : Outport  VectorParamsAs1DForOutWhenUnconnected=off
  wires:
  Bus Creator/1 -> Data/1  "EM_BOOT"
  raptor_can_rxmsg/2 -> CANRxField/1  "EM_BOOT_EmBoot"
  CANRxMsgStatus/1 -> Bus Creator/1
  DiagEnbl/1 -> CANRxMsgStatus/1
  raptor_can_rxmsg/1 -> CANRxMsgStatus/2  "Age"
  CANRxField/1 -> Bus Creator/2

== system VCMGCM1962020b_v2/Fgnd/Sensors/CAN/Inverter/MsgName ==
  DiagEnbl : Inport
  Bus Creator : BusCreator  Inputs=2
  CANRxField : Blocks_lib/CANRxField  typ='double'  custom=off  custom_nam='---'  custom_units='---'
  CANRxMsgStatus : Blocks_lib/CANRxMsgStatus  samptime=samptime  custom=off  custom_nam='Name'  msgnam=EM2
  Header : Blocks_lib/Header  width=Landscape  addtext=''
  raptor_can_rxmsg : Raptor_lib/CAN/raptor_can_rxmsg  canDefinition=struct('dbcFile', '20220526e_emDrive_NodeID_0x01.dbc','message', 'EM2','comment', '500ms','signals', {{'EM2_InverterBridgeMaxTemp','EM2_MotorSensorTemp'}},'enabled', [ 1 1;],'scaled', [ 1 1;],'canBus', 'bus','messageID', [ 1153;],'idMask', [ 536870911;],'payloadMask', [],'payloadValue', [],'period', [ 0;],'mailbox', '''''','queueSize', [ 1;],'label', [ 1;],'ver', [ 2;],'showID', [ 0;],'showRaw', [ 0;],'fill', [ 0;],'editID', [ 0;],'signalOrder', [ 3;],'signalAscDes', [ 1;])  canBus=bus  mailbox=''  payloadMask=[]  payloadValue=[]  idMask=hex2dec('1FFFFFFF')  queueSize=1  showID=0  label=1  fill=0  id=1153  showRaw=0  showAge=1  signalOrder=3  signalInfo={{struct('Name', 'EM2_InverterBridgeMaxTemp','Startbit', [ 0;],'SignalSize', [ 32;],'ByteOrder', 'LittleEndian','ValueType', 'FLOAT32','Class', 'single','Signed', [ 1;],'Factor', [ 1;],'Offset', [ 0;],'Min', [ -50;],'Max', [ 250;],'Units', 'degC','Comment', 'Ctrl_Bridge_StatusMaxTemp','StartBit', [ 0;]),struct('Name', 'EM2_MotorSensorTemp','Startbit', [ 0;],'SignalSize', [ 32;],'ByteOrder', 'LittleEndian','ValueType', 'FLOAT32','Class', 'single','Signed', [ 1;],'Factor', [ 1;],'Offset', [ 0;],'Min', [ -50;],'Max', [ 250;],'Units', 'degC','Comment', 'Ctrl_Gen_Stat__MotorSensorTemp','StartBit', [ 32;])}}
      settings: SourceProductName=Raptor
  Data : Outport  VectorParamsAs1DForOutWhenUnconnected=off
  wires:
  CANRxField/1 -> Bus Creator/2
  raptor_can_rxmsg/1 -> CANRxMsgStatus/2  "Age"
  DiagEnbl/1 -> CANRxMsgStatus/1
  CANRxMsgStatus/1 -> Bus Creator/1
  raptor_can_rxmsg/2 -> CANRxField/1  "EM2_InverterBridgeMaxTemp"
  Bus Creator/1 -> Data/1  "MsgName"

== system VCMGCM1962020b_v2/Fgnd/Sensors/CAN/Other/A//C Compressor ==
  Data : Inport
  ACCSTATUS2 : Subsystem  mask{samptime=samptime}
      mask prompts: samptime "Sample Time (sec)"
      mask help:
      | Example of how to set up a CAN message recieve.
      | 1. Copy this block into the main model.
      | 2. Disable/break library link.
      | 3. Underneath, set up CAN Rx Message block.
      | 4. For each field, connect a CANRxField block from the CAN block to the bus creator; adjust parameters as necessary.
      mask init:
      | [msgnam, msgbus] = CANBlockInit('Rx');
      mask Display: disp(['CAN Rx: Message\n' msgnam '\n' msgbus]);
  Bus Creator : BusCreator  Inputs=2
  Bus Selector : BusSelector  OutputSignals=Control.Other.Other.SysWake [Bool]
  CANRxDiagEnbl : Blocks_lib/CANRxDiagEnbl  nam=nam
  Header : Blocks_lib/Header  width=Portrait  addtext=''
  MsgName : Subsystem  mask{samptime=samptime}
      mask prompts: samptime "Sample Time (sec)"
      mask help:
      | Example of how to set up a CAN message recieve.
      | 1. Copy this block into the main model.
      | 2. Disable/break library link.
      | 3. Underneath, set up CAN Rx Message block.
      | 4. For each field, connect a CANRxField block from the CAN block to the bus creator; adjust parameters as necessary.
      mask init:
      | [msgnam, msgbus] = CANBlockInit('Rx');
      mask Display: disp(['CAN Rx: Message\n' msgnam '\n' msgbus]);
  CAN : Outport  VectorParamsAs1DForOutWhenUnconnected=off
  wires:
  CANRxDiagEnbl/1 -> ACCSTATUS2/1(DiagEnbl), MsgName/1(DiagEnbl)
  Bus Selector/1 -> CANRxDiagEnbl/1  "<SysWake [Bool]>"
  Bus Creator/1 -> CAN/1  "ACC"
  Data/1 -> Bus Selector/1
  ACCSTATUS2/1(Data) -> Bus Creator/2
  MsgName/1(Data) -> Bus Creator/1

== system VCMGCM1962020b_v2/Fgnd/Sensors/CAN/Other/BCM ==
  Data : Inport
  BCMAMB : Subsystem  mask{samptime=samptime}
      mask prompts: samptime "Sample Time (sec)"
      mask help:
      | Example of how to set up a CAN message recieve.
      | 1. Copy this block into the main model.
      | 2. Disable/break library link.
      | 3. Underneath, set up CAN Rx Message block.
      | 4. For each field, connect a CANRxField block from the CAN block to the bus creator; adjust parameters as necessary.
      mask init:
      | [msgnam, msgbus] = CANBlockInit('Rx');
      mask Display: disp(['CAN Rx: Message\n' msgnam '\n' msgbus]);
  BCMCab_Mssg1 : Subsystem  mask{samptime=samptime}
      mask prompts: samptime "Sample Time (sec)"
      mask help:
      | Example of how to set up a CAN message recieve.
      | 1. Copy this block into the main model.
      | 2. Disable/break library link.
      | 3. Underneath, set up CAN Rx Message block.
      | 4. For each field, connect a CANRxField block from the CAN block to the bus creator; adjust parameters as necessary.
      mask init:
      | [msgnam, msgbus] = CANBlockInit('Rx');
      mask Display: disp(['CAN Rx: Message\n' msgnam '\n' msgbus]);
  Bus Creator : BusCreator  Inputs=3
  Bus Selector : BusSelector  OutputSignals=Control.Mode.StartStop.OutptDiagEnbl [Bool]
  CANRxDiagEnbl : Blocks_lib/CANRxDiagEnbl  nam=nam
  CCVS1_BCM : Subsystem  mask{samptime=samptime}
      mask prompts: samptime "Sample Time (sec)"
      mask help:
      | Example of how to set up a CAN message recieve.
      | 1. Copy this block into the main model.
      | 2. Disable/break library link.
      | 3. Underneath, set up CAN Rx Message block.
      | 4. For each field, connect a CANRxField block from the CAN block to the bus creator; adjust parameters as necessary.
      mask init:
      | [msgnam, msgbus] = CANBlockInit('Rx');
      mask Display: disp(['CAN Rx: Message\n' msgnam '\n' msgbus]);
  Header : Blocks_lib/Header  width=Portrait  addtext=''
  CAN : Outport  VectorParamsAs1DForOutWhenUnconnected=off
  wires:
  Bus Creator/1 -> CAN/1  "BCM"
  BCMAMB/1(Data) -> Bus Creator/1
  CCVS1_BCM/1(Data) -> Bus Creator/2
  Data/1 -> Bus Selector/1
  Bus Selector/1 -> CANRxDiagEnbl/1  "<OutptDiagEnbl [Bool]>"
  CANRxDiagEnbl/1 -> BCMCab_Mssg1/1(DiagEnbl), CCVS1_BCM/1(DiagEnbl), BCMAMB/1(DiagEnbl)
  BCMCab_Mssg1/1(Data) -> Bus Creator/3

== system VCMGCM1962020b_v2/Fgnd/Sensors/CAN/Other/BCM1 ==
  Data : Inport
  Bus Creator : BusCreator  Inputs=1
  Bus Selector : BusSelector  OutputSignals=Control.Mode.StartStop.CANDiagEnbl [Bool]
  CANRxDiagEnbl : Blocks_lib/CANRxDiagEnbl  nam=nam
  DisplayTG1 : Subsystem  mask{samptime=samptime}
      mask prompts: samptime "Sample Time (sec)"
      mask help:
      | Example of how to set up a CAN message recieve.
      | 1. Copy this block into the main model.
      | 2. Disable/break library link.
      | 3. Underneath, set up CAN Rx Message block.
      | 4. For each field, connect a CANRxField block from the CAN block to the bus creator; adjust parameters as necessary.
      mask init:
      | [msgnam, msgbus] = CANBlockInit('Rx');
      mask Display: disp(['CAN Rx: Message\n' msgnam '\n' msgbus]);
  Header : Blocks_lib/Header  width=Portrait  addtext=''
  CAN : Outport  VectorParamsAs1DForOutWhenUnconnected=off
  wires:
  Bus Creator/1 -> CAN/1  "Display"
  DisplayTG1/1(Data) -> Bus Creator/1
  Data/1 -> Bus Selector/1
  Bus Selector/1 -> CANRxDiagEnbl/1  "<CANDiagEnbl [Bool]>"
  CANRxDiagEnbl/1 -> DisplayTG1/1(DiagEnbl)

== system VCMGCM1962020b_v2/Fgnd/Sensors/CAN/Other/Charge Port DC Voltage Sensor ==
  Data : Inport
  Bus Creator : BusCreator  Inputs=1
  Bus Selector : BusSelector  OutputSignals=Control.Mode.StartStop.CANDiagEnbl [Bool]
  Header : Blocks_lib/Header  width=Portrait  addtext=''
  cs_ivt_msg_result_voltage_ch1 : Subsystem  mask{samptime=samptime}
      mask prompts: samptime "Sample Time (sec)"
      mask help:
      | Example of how to set up a CAN message recieve.
      | 1. Copy this block into the main model.
      | 2. Disable/break library link.
      | 3. Underneath, set up CAN Rx Message block.
      | 4. For each field, connect a CANRxField block from the CAN block to the bus creator; adjust parameters as necessary.
      mask init:
      | [msgnam, msgbus] = CANBlockInit('Rx');
      mask Display: disp(['CAN Rx: Message\n' msgnam '\n' msgbus]);
  CAN : Outport  VectorParamsAs1DForOutWhenUnconnected=off
  wires:
  Bus Creator/1 -> CAN/1  "ChgPortDCVolt"
  Data/1 -> Bus Selector/1
  cs_ivt_msg_result_voltage_ch1/1(Data) -> Bus Creator/1
  Bus Selector/1 -> cs_ivt_msg_result_voltage_ch1/1(DiagEnbl)  "<CANDiagEnbl [Bool]>"

== system VCMGCM1962020b_v2/Fgnd/Sensors/CAN/Other/Cooling Pump 1 ==
  Data : Inport
  Bus Creator : BusCreator  Inputs=2
  Bus Selector : BusSelector  OutputSignals=Control.Other.Other.SysWake [Bool]
  CANRxDiagEnbl : Blocks_lib/CANRxDiagEnbl  nam=nam
  CANRxJ1939DM1(w/oTP) : Blocks_lib/CANRxJ1939DM1(w//oTP)  nam=nam  bus=bus  samptime=samptime
  Header : Blocks_lib/Header  width=Portrait  addtext=''
  MsgName : Subsystem  mask{samptime=samptime}
      mask prompts: samptime "Sample Time (sec)"
      mask help:
      | Example of how to set up a CAN message recieve.
      | 1. Copy this block into the main model.
      | 2. Disable/break library link.
      | 3. Underneath, set up CAN Rx Message block.
      | 4. For each field, connect a CANRxField block from the CAN block to the bus creator; adjust parameters as necessary.
      mask init:
      | [msgnam, msgbus] = CANBlockInit('Rx');
      mask Display: disp(['CAN Rx: Message\n' msgnam '\n' msgbus]);
  Set Rx IDs : Subsystem
  raptor_app_trigger : Raptor_lib/Triggers/raptor_app_trigger  triggerValues=Startup|Shutdown|SafetyMonitor  trigger=Startup  inherited=1  alwaysEnabled=1  triggerPriority=0  triggerName=Startup_P09ht  allowInline=0
      settings: SourceProductName=Raptor
  CAN : Outport  VectorParamsAs1DForOutWhenUnconnected=off
  wires:
  CANRxJ1939DM1(w/oTP)/1 -> Bus Creator/2
  raptor_app_trigger/1 -> Set Rx IDs/Trigger
  Bus Creator/1 -> CAN/1  "CoolPump1"
  MsgName/1(Data) -> Bus Creator/1
  Data/1 -> Bus Selector/1
  Bus Selector/1 -> CANRxDiagEnbl/1  "<SysWake [Bool]>"
  CANRxDiagEnbl/1 -> CANRxJ1939DM1(w/oTP)/1, MsgName/1(DiagEnbl)

== system VCMGCM1962020b_v2/Fgnd/Sensors/CAN/Other/Cooling Pump 2 ==
  Data : Inport
  Bus Creator : BusCreator  Inputs=2
  Bus Selector : BusSelector  OutputSignals=Control.Other.Other.SysWake [Bool]
  CANRxDiagEnbl : Blocks_lib/CANRxDiagEnbl  nam=nam
  CANRxJ1939DM1(w/oTP) : Blocks_lib/CANRxJ1939DM1(w//oTP)  nam=nam  bus=bus  samptime=samptime
  Header : Blocks_lib/Header  width=Portrait  addtext=''
  MsgName : Subsystem  mask{samptime=samptime}
      mask prompts: samptime "Sample Time (sec)"
      mask help:
      | Example of how to set up a CAN message recieve.
      | 1. Copy this block into the main model.
      | 2. Disable/break library link.
      | 3. Underneath, set up CAN Rx Message block.
      | 4. For each field, connect a CANRxField block from the CAN block to the bus creator; adjust parameters as necessary.
      mask init:
      | [msgnam, msgbus] = CANBlockInit('Rx');
      mask Display: disp(['CAN Rx: Message\n' msgnam '\n' msgbus]);
  Set Rx IDs : Subsystem
  raptor_app_trigger : Raptor_lib/Triggers/raptor_app_trigger  triggerValues=Startup|Shutdown|SafetyMonitor  trigger=Startup  inherited=1  alwaysEnabled=1  triggerPriority=0  triggerName=Startup_Rn9p7  allowInline=0
      settings: SourceProductName=Raptor
  CAN : Outport  VectorParamsAs1DForOutWhenUnconnected=off
  wires:
  CANRxDiagEnbl/1 -> MsgName/1(DiagEnbl), CANRxJ1939DM1(w/oTP)/1
  Bus Selector/1 -> CANRxDiagEnbl/1  "<SysWake [Bool]>"
  Data/1 -> Bus Selector/1
  MsgName/1(Data) -> Bus Creator/1
  Bus Creator/1 -> CAN/1  "CoolPump2"
  raptor_app_trigger/1 -> Set Rx IDs/Trigger
  CANRxJ1939DM1(w/oTP)/1 -> Bus Creator/2

== system VCMGCM1962020b_v2/Fgnd/Sensors/CAN/Other/EPAS ==
  Data : Inport
  Bus Creator : BusCreator  Inputs=10
  Bus Selector : BusSelector  OutputSignals=Control.Mode.StartStop.CANDiagEnbl [Bool]
  CANRxDiagEnbl : Blocks_lib/CANRxDiagEnbl  nam=nam
  EPASG7GenericFdbk0 : Subsystem  mask{samptime=samptime}
      mask prompts: samptime "Sample Time (sec)"
      mask help:
      | Example of how to set up a CAN message recieve.
      | 1. Copy this block into the main model.
      | 2. Disable/break library link.
      | 3. Underneath, set up CAN Rx Message block.
      | 4. For each field, connect a CANRxField block from the CAN block to the bus creator; adjust parameters as necessary.
      mask init:
      | [msgnam, msgbus] = CANBlockInit('Rx');
      mask Display: disp(['CAN Rx: Message\n' msgnam '\n' msgbus]);
  EPASG7GenericFdbk1 : Subsystem  mask{samptime=samptime}
      mask prompts: samptime "Sample Time (sec)"
      mask help:
      | Example of how to set up a CAN message recieve.
      | 1. Copy this block into the main model.
      | 2. Disable/break library link.
      | 3. Underneath, set up CAN Rx Message block.
      | 4. For each field, connect a CANRxField block from the CAN block to the bus creator; adjust parameters as necessary.
      mask init:
      | [msgnam, msgbus] = CANBlockInit('Rx');
      mask Display: disp(['CAN Rx: Message\n' msgnam '\n' msgbus]);
  EPASG7GenericFdbk2 : Subsystem  mask{samptime=samptime}
      mask prompts: samptime "Sample Time (sec)"
      mask help:
      | Example of how to set up a CAN message recieve.
      | 1. Copy this block into the main model.
      | 2. Disable/break library link.
      | 3. Underneath, set up CAN Rx Message block.
      | 4. For each field, connect a CANRxField block from the CAN block to the bus creator; adjust parameters as necessary.
      mask init:
      | [msgnam, msgbus] = CANBlockInit('Rx');
      mask Display: disp(['CAN Rx: Message\n' msgnam '\n' msgbus]);
  EPASG7GenericFdbk3 : Subsystem  mask{samptime=samptime}
      mask prompts: samptime "Sample Time (sec)"
      mask help:
      | Example of how to set up a CAN message recieve.
      | 1. Copy this block into the main model.
      | 2. Disable/break library link.
      | 3. Underneath, set up CAN Rx Message block.
      | 4. For each field, connect a CANRxField block from the CAN block to the bus creator; adjust parameters as necessary.
      mask init:
      | [msgnam, msgbus] = CANBlockInit('Rx');
      mask Display: disp(['CAN Rx: Message\n' msgnam '\n' msgbus]);
  EPASG7GenericFdbk4 : Subsystem  mask{samptime=samptime}
      mask prompts: samptime "Sample Time (sec)"
      mask help:
      | Example of how to set up a CAN message recieve.
      | 1. Copy this block into the main model.
      | 2. Disable/break library link.
      | 3. Underneath, set up CAN Rx Message block.
      | 4. For each field, connect a CANRxField block from the CAN block to the bus creator; adjust parameters as necessary.
      mask init:
      | [msgnam, msgbus] = CANBlockInit('Rx');
      mask Display: disp(['CAN Rx: Message\n' msgnam '\n' msgbus]);
  EPASG7GenericFdbk6 : Subsystem  mask{samptime=samptime}
      mask prompts: samptime "Sample Time (sec)"
      mask help:
      | Example of how to set up a CAN message recieve.
      | 1. Copy this block into the main model.
      | 2. Disable/break library link.
      | 3. Underneath, set up CAN Rx Message block.
      | 4. For each field, connect a CANRxField block from the CAN block to the bus creator; adjust parameters as necessary.
      mask init:
      | [msgnam, msgbus] = CANBlockInit('Rx');
      mask Display: disp(['CAN Rx: Message\n' msgnam '\n' msgbus]);
  EPASG7GenericFdbk7 : Subsystem  mask{samptime=samptime}
      mask prompts: samptime "Sample Time (sec)"
      mask help:
      | Example of how to set up a CAN message recieve.
      | 1. Copy this block into the main model.
      | 2. Disable/break library link.
      | 3. Underneath, set up CAN Rx Message block.
      | 4. For each field, connect a CANRxField block from the CAN block to the bus creator; adjust parameters as necessary.
      mask init:
      | [msgnam, msgbus] = CANBlockInit('Rx');
      mask Display: disp(['CAN Rx: Message\n' msgnam '\n' msgbus]);
  EPASG7GenericFdbk8 : Subsystem  mask{samptime=samptime}
      mask prompts: samptime "Sample Time (sec)"
      mask help:
      | Example of how to set up a CAN message recieve.
      | 1. Copy this block into the main model.
      | 2. Disable/break library link.
      | 3. Underneath, set up CAN Rx Message block.
      | 4. For each field, connect a CANRxField block from the CAN block to the bus creator; adjust parameters as necessary.
      mask init:
      | [msgnam, msgbus] = CANBlockInit('Rx');
      mask Display: disp(['CAN Rx: Message\n' msgnam '\n' msgbus]);
  EPASG7GenericFdbk9 : Subsystem  mask{samptime=samptime}
      mask prompts: samptime "Sample Time (sec)"
      mask help:
      | Example of how to set up a CAN message recieve.
      | 1. Copy this block into the main model.
      | 2. Disable/break library link.
      | 3. Underneath, set up CAN Rx Message block.
      | 4. For each field, connect a CANRxField block from the CAN block to the bus creator; adjust parameters as necessary.
      mask init:
      | [msgnam, msgbus] = CANBlockInit('Rx');
      mask Display: disp(['CAN Rx: Message\n' msgnam '\n' msgbus]);
  Header : Blocks_lib/Header  width=Portrait  addtext=''
  CAN : Outport  VectorParamsAs1DForOutWhenUnconnected=off
  wires:
  CANRxDiagEnbl/1 -> EPASG7GenericFdbk9/1(DiagEnbl), EPASG7GenericFdbk8/1(DiagEnbl), EPASG7GenericFdbk7/1(DiagEnbl), EPASG7GenericFdbk6/1(DiagEnbl), EPASG7GenericFdbk4/1(DiagEnbl), EPASG7GenericFdbk3/1(DiagEnbl), EPASG7GenericFdbk2/1(DiagEnbl), EPASG7GenericFdbk1/1(DiagEnbl), EPASG7GenericFdbk0/1(DiagEnbl)
  Bus Selector/1 -> CANRxDiagEnbl/1  "<CANDiagEnbl [Bool]>"
  Data/1 -> Bus Selector/1
  Bus Creator/1 -> CAN/1  "EPAS"
  EPASG7GenericFdbk0/1(Data) -> Bus Creator/2
  EPASG7GenericFdbk1/1(Data) -> Bus Creator/3
  EPASG7GenericFdbk2/1(Data) -> Bus Creator/4
  EPASG7GenericFdbk3/1(Data) -> Bus Creator/5
  EPASG7GenericFdbk4/1(Data) -> Bus Creator/6
  EPASG7GenericFdbk6/1(Data) -> Bus Creator/7
  EPASG7GenericFdbk7/1(Data) -> Bus Creator/8
  EPASG7GenericFdbk8/1(Data) -> Bus Creator/9
  EPASG7GenericFdbk9/1(Data) -> Bus Creator/10

== system VCMGCM1962020b_v2/Fgnd/Sensors/CAN/Other/Heater ==
  Data : Inport
  Bus Creator : BusCreator  Inputs=2
  Bus Selector : BusSelector  OutputSignals=Control.Other.Other.SysWake [Bool]
  CANRxDiagEnbl : Blocks_lib/CANRxDiagEnbl  nam='Heater'
  HTR_OUT_2 : Subsystem  mask{samptime=samptime}
      mask prompts: samptime "Sample Time (sec)"
      mask help:
      | Example of how to set up a CAN message recieve.
      | 1. Copy this block into the main model.
      | 2. Disable/break library link.
      | 3. Underneath, set up CAN Rx Message block.
      | 4. For each field, connect a CANRxField block from the CAN block to the bus creator; adjust parameters as necessary.
      mask init:
      | [msgnam, msgbus] = CANBlockInit('Rx');
      mask Display: disp(['CAN Rx: Message\n' msgnam '\n' msgbus]);
  Header : Blocks_lib/Header  width=Portrait  addtext=''
  MsgName : Subsystem  mask{samptime=samptime}
      mask prompts: samptime "Sample Time (sec)"
      mask help:
      | Example of how to set up a CAN message recieve.
      | 1. Copy this block into the main model.
      | 2. Disable/break library link.
      | 3. Underneath, set up CAN Rx Message block.
      | 4. For each field, connect a CANRxField block from the CAN block to the bus creator; adjust parameters as necessary.
      mask init:
      | [msgnam, msgbus] = CANBlockInit('Rx');
      mask Display: disp(['CAN Rx: Message\n' msgnam '\n' msgbus]);
  CAN : Outport  VectorParamsAs1DForOutWhenUnconnected=off
  wires:
  Bus Selector/1 -> CANRxDiagEnbl/1  "<SysWake [Bool]>"
  Bus Creator/1 -> CAN/1  "Heater"
  Data/1 -> Bus Selector/1
  HTR_OUT_2/1(Data) -> Bus Creator/2
  MsgName/1(Data) -> Bus Creator/1
  CANRxDiagEnbl/1 -> MsgName/1(DiagEnbl), HTR_OUT_2/1(DiagEnbl)

== system VCMGCM1962020b_v2/Fgnd/Sensors/CAN/Other/Power Steering Pump Inverter ==
  Data : Inport
  Bus Creator : BusCreator  Inputs=4
  Bus Selector : BusSelector  OutputSignals=Control.Other.Other.SysWake [Bool]
  CANRxDiagEnbl : Blocks_lib/CANRxDiagEnbl  nam=nam
  Header : Blocks_lib/Header  width=Portrait  addtext=''
  MsgName : Subsystem  mask{samptime=samptime}
      mask prompts: samptime "Sample Time (sec)"
      mask help:
      | Example of how to set up a CAN message recieve.
      | 1. Copy this block into the main model.
      | 2. Disable/break library link.
      | 3. Underneath, set up CAN Rx Message block.
      | 4. For each field, connect a CANRxField block from the CAN block to the bus creator; adjust parameters as necessary.
      mask init:
      | [msgnam, msgbus] = CANBlockInit('Rx');
      mask Display: disp(['CAN Rx: Message\n' msgnam '\n' msgbus]);
  PSPInvtrHS2_Status_Feedback : Subsystem  mask{samptime=samptime}
      mask prompts: samptime "Sample Time (sec)"
      mask help:
      | Example of how to set up a CAN message recieve.
      | 1. Copy this block into the main model.
      | 2. Disable/break library link.
      | 3. Underneath, set up CAN Rx Message block.
      | 4. For each field, connect a CANRxField block from the CAN block to the bus creator; adjust parameters as necessary.
      mask init:
      | [msgnam, msgbus] = CANBlockInit('Rx');
      mask Display: disp(['CAN Rx: Message\n' msgnam '\n' msgbus]);
  PSPInvtrHS3_Temperature_Feedback : Subsystem  mask{samptime=samptime}
      mask prompts: samptime "Sample Time (sec)"
      mask help:
      | Example of how to set up a CAN message recieve.
      | 1. Copy this block into the main model.
      | 2. Disable/break library link.
      | 3. Underneath, set up CAN Rx Message block.
      | 4. For each field, connect a CANRxField block from the CAN block to the bus creator; adjust parameters as necessary.
      mask init:
      | [msgnam, msgbus] = CANBlockInit('Rx');
      mask Display: disp(['CAN Rx: Message\n' msgnam '\n' msgbus]);
  PSPInvtrHS4_Fault_Info : Subsystem  mask{samptime=samptime}
      mask prompts: samptime "Sample Time (sec)"
      mask help:
      | Example of how to set up a CAN message recieve.
      | 1. Copy this block into the main model.
      | 2. Disable/break library link.
      | 3. Underneath, set up CAN Rx Message block.
      | 4. For each field, connect a CANRxField block from the CAN block to the bus creator; adjust parameters as necessary.
      mask init:
      | [msgnam, msgbus] = CANBlockInit('Rx');
      mask Display: disp(['CAN Rx: Message\n' msgnam '\n' msgbus]);
  Set Rx IDs : Subsystem
  raptor_app_trigger : Raptor_lib/Triggers/raptor_app_trigger  triggerValues=Startup|Shutdown|SafetyMonitor  trigger=Startup  inherited=1  alwaysEnabled=1  triggerPriority=0  triggerName=Startup_XK4fp  allowInline=0
      settings: SourceProductName=Raptor
  CAN : Outport  VectorParamsAs1DForOutWhenUnconnected=off
  wires:
  raptor_app_trigger/1 -> Set Rx IDs/Trigger
  Bus Creator/1 -> CAN/1  "PSPInvtr"
  MsgName/1(Data) -> Bus Creator/1
  PSPInvtrHS2_Status_Feedback/1(Data) -> Bus Creator/2
  PSPInvtrHS3_Temperature_Feedback/1(Data) -> Bus Creator/3
  PSPInvtrHS4_Fault_Info/1(Data) -> Bus Creator/4
  Data/1 -> Bus Selector/1
  Bus Selector/1 -> CANRxDiagEnbl/1  "<SysWake [Bool]>"
  CANRxDiagEnbl/1 -> MsgName/1(DiagEnbl), PSPInvtrHS2_Status_Feedback/1(DiagEnbl), PSPInvtrHS3_Temperature_Feedback/1(DiagEnbl), PSPInvtrHS4_Fault_Info/1(DiagEnbl)
